simulink model "project_milestone_4"  (R2016a)
settings: Solver=VariableStepAuto  StartTime=0.0  StopTime=10.0  RelTol=1e-3
undefined symbols (not defined in the file): Radix
libraries: simulink x2, dspspect3 x1, dsparch4 x1
settings Model: Creator=Raj  LastModifiedBy=Raj

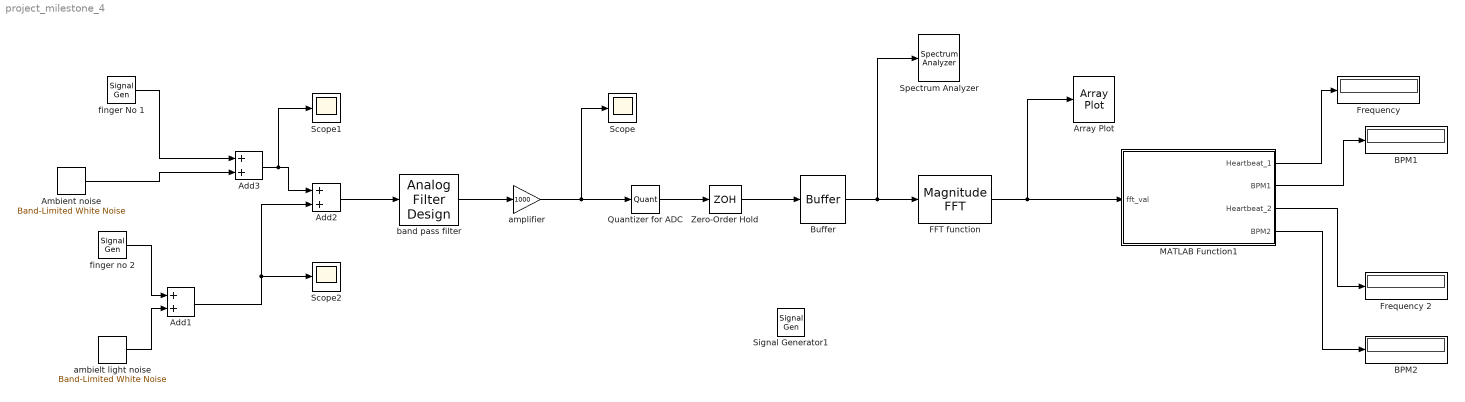
== system project_milestone_4 ==
  Add1 : Sum
  Add2 : Sum
  Add3 : Sum
  "Ambient noise " : simulink/Sources/Band-Limited White Noise  Cov=1e-7  Ts=0.001  seed=[23341]
  Array Plot : ArrayPlot
  BPM1 : Display
  BPM2 : Display
  Buffer : Buffer  N=1024  TreatMby1Signals=One channel  OutputFrames=off
  FFT function : dspspect3/Magnitude FFT  mag_or_magsq=Magnitude  FFTImplementation=Radix-2  fftLenInherit=off  fftsize=1024  WrapInput=on
  Frequency : Display
  Frequency 2 : Display
  MATLAB Function1 : MATLAB Function  TreatAsAtomicUnit=on
  Quantizer for ADC : Quantizer  QuantizationInterval=0.005
  Scope : Scope
  Scope1 : Scope
  Scope2 : Scope
  Signal Generator1 : SignalGenerator  Units=rad/sec
  Spectrum Analyzer : SpectrumAnalyzer
  Zero-Order Hold : ZeroOrderHold  SampleTime=0.005
  "ambielt light noise " : simulink/Sources/Band-Limited White Noise  Cov=1e-7  Ts=0.001  seed=[23341]
  "amplifier " : Gain  Gain=1000
  "band pass filter " : dsparch4/Analog Filter Design  method=Butterworth  filttype=Bandpass  N=1  Wlo=3.14  Whi=15.71  Rp=2  Rs=40
  "finger No 1 " : SignalGenerator  WaveForm=sawtooth  Amplitude=0.020  Frequency=1.5
  "finger no 2 " : SignalGenerator  WaveForm=sawtooth  Amplitude=0.020  Frequency=2
  wires:
  "finger no 2 "/1 -> Add1/1
  "ambielt light noise "/1 -> Add1/2
  Add2/1 -> "band pass filter "/1
  "band pass filter "/1 -> "amplifier "/1
  "amplifier "/1 -> Scope/1, Quantizer for ADC/1
  Add1/1 -> Scope2/1, Add2/2
  Quantizer for ADC/1 -> Zero-Order Hold/1
  Zero-Order Hold/1 -> Buffer/1
  Buffer/1 -> Spectrum Analyzer/1, FFT function/1
  FFT function/1 -> Array Plot/1, MATLAB Function1/1(fft_val)
  MATLAB Function1/1(Heartbeat_1) -> Frequency/1
  MATLAB Function1/3(Heartbeat_2) -> Frequency 2/1
  MATLAB Function1/2(BPM1) -> BPM1/1
  MATLAB Function1/4(BPM2) -> BPM2/1
  Add3/1 -> Scope1/1, Add2/1
  "Ambient noise "/1 -> Add3/2
  "finger No 1 "/1 -> Add3/1

== matlab function project_milestone_4/MATLAB Function1 ==
  data: fft_val input; Heartbeat_1 output; BPM1 output; Heartbeat_2 output; BPM2 output
function [ Heartbeat_1 ,BPM1 , Heartbeat_2 ,  BPM2 ] = fcn(fft_val )
%#codegen
[no1, pos1] = max(fft_val(4 : 24));
fft_val(pos1+3) = 0; 
[no2 , pos2]= max(fft_val(4 : 24));

val_1= pos1+2;
val_2 =  pos2+2;

Heartbeat_1= ((200/1024)*(pos1+2));
BPM1 = Heartbeat_1*60;
Heartbeat_2= ((200/1024)*(pos2+2));
BPM2 = Heartbeat_2*60;
